simulink model "ACC_Example"  (R2015a)
settings: Solver=ode3  StartTime=0.0  StopTime=2000  FixedStep=0.02  RelTol=1e-3
undefined symbols (not defined in the file): control, data, serial
libraries: simulink x14, dspsigops x8, simulink_extras x4, instrumentlib x4, dspswit3 x1
settings Model: SimulationMode=accelerator  CovSFcnEnable=off  Creator=Owen  LastModifiedBy=VijayaKumar
settings OptimizationCC: EfficientMapNaN2IntZero=off  AccelVerboseBuild=on
settings DebuggingCC: SolverPrmCheckMsg=warning
settings HardwareCC: TargetLongLongMode=on  TargetIntDivRoundTo=Zero  TargetEndianess=LittleEndian  TargetHWDeviceType=MATLAB Host  ProdEqTarget=off
settings SFSimCC: SimCustomInitializer=initTORCSLink();  SimCustomTerminator=terminateTORCSLink();  SimUserSources=TORCSLink.c  SimBuildMode=sf_nonincremental_build  SimGenImportedTypeDefs=on
settings CodeAppCC: MaxIdLength=128
settings GRTTargetCC: CombineOutputUpdateFcns=off  GRTInterface=on

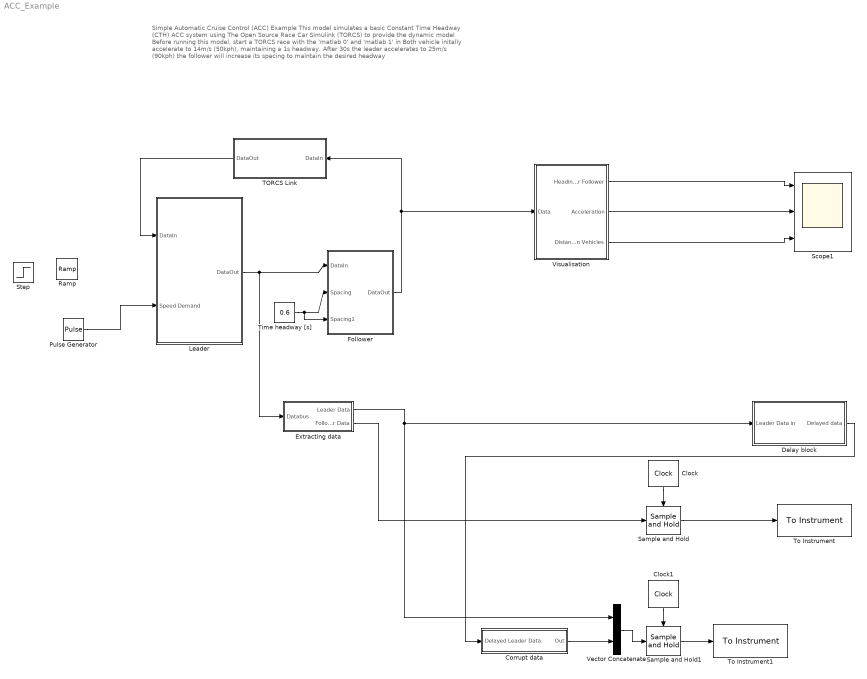
== system ACC_Example ==
  note: Simple Automatic Cruise Control (ACC) Example
      |
      | This model simulates a basic Constant Time Headway (CTH) ACC system using
      | The Open Source Race Car Simulink (TORCS) to provide the dynamic model
      |
      | Before running this model, start a TORCS race with the 'matlab 0' and 'matlab 1' in
      |
      | Both vehicle initally accelerate to 14m/s (50kph), maintaining a 1s headway.
      | After 30s the leader accelerates to 25m/s (90kph)
      | the follower will increase its spacing to maintain the desired headway
  Clock : simulink_extras/Flip Flops/Clock  period=0.04
  Clock1 : simulink_extras/Flip Flops/Clock  period=0.04
  Corrupt data : Subsystem
  "Delay block " : Subsystem
  Extracting data : Subsystem
  Follower : Subsystem
      settings: CopyFcn=|
      | veh = str2num(get_param(gcb, 'vehicle'));
      | veh = veh + 1;
      | set_param(gcb,'vehicle',num2str(veh));
  Leader : Subsystem
  Pulse Generator : DiscretePulseGenerator  PulseType=Time based  Amplitude=25  Period=60  PulseWidth=95
  Ramp : simulink/Sources/Ramp  slope=0.01  start=0  X0=15
  Sample and Hold : dspsigops/Sample and Hold  trig=Rising edge  initCond=0  latchinput=off
  Sample and Hold1 : dspsigops/Sample and Hold  trig=Rising edge  initCond=0  latchinput=off
  Scope1 : Scope  NumInputPorts=3
      settings: YMin=-0.5~-20~-2000  YMax=0.2~25~500  MaxDataPoints=30000
  Step : Step  Time=15  Before=10  After=15  SampleTime=0
  TORCS Link : Subsystem  LoadFcn=|  InitFcn=|
      LoadFcn=|
      | load VehicleBusses.mat;
      | src = 'TORCSLink.c';
      | init = 'initTORCSLink();';
      | term = 'terminateTORCSLink();';
      | simSrc = get_param(gcs,'SimUserSources');
      | simInit = get_param(gcs,'SimCustomInitializer');
      | simTerm = get_param(gcs,'SimCustomTerminator');
      | 
      | if isempty(strfind(simSrc,src))
      |   fprintf('Adding %s to Custom Sources\n', src);
      |   set_param(gcs,'SimUserSources', [simSrc 10 src]);
      | end
      | 
      | if isempty(strfind(simInit,init))
      |   fprintf('Adding %s to Custom Initialisation Code\n', init);
      |   set_param(gcs,'SimCustomInitializer', [simInit 10 init]);
      | end
      | 
      | if isempty(strfind(simTerm,term))
      |   fprintf('Adding %s to Custom Termination Code\n', term);
      |   set_param(gcs,'SimCustomTerminator', [simTerm 10 term]);
      | end
      | 
      | if isunix
      |     libs = 'librt.so';
      |     simLibs = get_param(gcs,'SimUserLibraries');
      | 
      |     if isempty(strfind(simLibs,libs))
      |       fprintf('Adding %s to Custom Libraries\n', libs);
      |       set_param(gcs,'SimUserLibraries', [simLibs 10 libs]);
      |     end
      | else
      |    set_param(gcs,'SimUserLibraries', '');
      | end
      | 
      | clear src init term simSrc simInit simTerm libs simLibs;
      InitFcn=|
      | load VehicleBusses.mat;
      | src = 'TORCSLink.c';
      | init = 'initTORCSLink();';
      | term = 'terminateTORCSLink();';
      | simSrc = get_param(gcs,'SimUserSources');
      | simInit = get_param(gcs,'SimCustomInitializer');
      | simTerm = get_param(gcs,'SimCustomTerminator');
      | 
      | if isempty(strfind(simSrc,src))
      |   fprintf('Adding %s to Custom Sources\n', src);
      |   set_param(gcs,'SimUserSources', [simSrc 10 src]);
      | end
      | 
      | if isempty(strfind(simInit,init))
      |   fprintf('Adding %s to Custom Initialisation Code\n', init);
      |   set_param(gcs,'SimCustomInitializer', [simInit 10 init]);
      | end
      | 
      | if isempty(strfind(simTerm,term))
      |   fprintf('Adding %s to Custom Termination Code\n', term);
      |   set_param(gcs,'SimCustomTerminator', [simTerm 10 term]);
      | end
      | 
      | if isunix
      |     libs = 'librt.so';
      |     simLibs = get_param(gcs,'SimUserLibraries');
      | 
      |     if isempty(strfind(simLibs,libs))
      |       fprintf('Adding %s to Custom Libraries\n', libs);
      |       set_param(gcs,'SimUserLibraries', [simLibs 10 libs]);
      |     end
      | else
      |    set_param(gcs,'SimUserLibraries', '');
      | end
      | 
      | clear src init term simSrc simInit simTerm libs simLibs;
  Time headway [s] : Constant  Value=0.6
  To Instrument : instrumentlib/To Instrument  sampleTime=-1  isWorkspaceObject=off  timeout=10  inputBufferSize=1024  protocol=Serial  serialPort=COM1  baudRate=115200  gpibVendor=Agilent Technologies  boardIndex=0  primaryAddress=1  secondaryAddress=0  visaVendor=Agilent  visaSerialPort=0  chassisIndex=0  logicalAddress=0  tcpRemoteHost='127.0.0.1'  tcpRemotePort=4500  udpRemoteHost='127.0.0.1'  udpRemotePort=9090  visaTCPBoardIndex=0  visaTCPRemoteHost='127.0.0.1'  usbBoardIndex=0  usbManufID=0  usbModelCode=0  usbSerialNumber=0  initAction=None  initCommand='DATA:SOURCE CH1'  initFunction=get  command=''  sendFormat=Binary  asciiFormatting='%d'  precision=32-bit float  byteOrder=Big Endian
  To Instrument1 : instrumentlib/To Instrument  sampleTime=-1  isWorkspaceObject=off  timeout=10  inputBufferSize=1024  protocol=Serial  serialPort=COM4  baudRate=115200  gpibVendor=Agilent Technologies  boardIndex=0  primaryAddress=1  secondaryAddress=0  visaVendor=Agilent  visaSerialPort=0  chassisIndex=0  logicalAddress=0  tcpRemoteHost='127.0.0.1'  tcpRemotePort=4500  udpRemoteHost='127.0.0.1'  udpRemotePort=9090  visaTCPBoardIndex=0  visaTCPRemoteHost='127.0.0.1'  usbBoardIndex=0  usbManufID=0  usbModelCode=0  usbSerialNumber=0  initAction=None  initCommand='DATA:SOURCE CH1'  initFunction=get  command=''  sendFormat=Binary  asciiFormatting='%d'  precision=32-bit float  byteOrder=Big Endian
  Vector Concatenate : Concatenate
  Visualisation : Subsystem
  wires:
  Leader/1(DataOut) -> Extracting data/1(Databus), Follower/1(DataIn)
  TORCS Link/1(DataOut) -> Leader/1(DataIn)
  Time headway [s]/1 -> Follower/3(Spacing1), Follower/2(Spacing)
  Clock/1 -> Sample and Hold/Trigger
  Extracting data/2(Follower Data) -> Sample and Hold/1
  Extracting data/1(Leader Data) -> Vector Concatenate/1, "Delay block "/1(Leader Data in)
  Clock1/1 -> Sample and Hold1/Trigger
  Sample and Hold1/1 -> To Instrument1/1
  Vector Concatenate/1 -> Sample and Hold1/1
  Pulse Generator/1 -> Leader/2(Speed Demand)
  Visualisation/2(Acceleration) -> Scope1/2
  Visualisation/1(Heading Error Follower) -> Scope1/1
  "Delay block "/1(Delayed data) -> Corrupt data/1(Delayed Leader Data)
  Corrupt data/1(Out) -> Vector Concatenate/2
  Follower/1(DataOut) -> TORCS Link/1(DataIn), Visualisation/1(Data)
  Visualisation/3(Distance Between Vehicles) -> Scope1/3
  Sample and Hold/1 -> To Instrument/1

== system ACC_Example/Corrupt data ==
  Delayed Leader Data : Inport
  Clock2 : simulink_extras/Flip Flops/Clock  period=0.04
  Constant{,1..3} (4 alike) : Constant  Value=2
  Counter : dspswit3/Counter  Direction=Up  CountEvent=Rising edge  CounterSize=User defined  MaxCount=255  InitialCount=0  Output=Count and Hit  HitValue=0  ResetInput=on  SamplesPerFrame=1  Ts=1  CntDtype=double  HitDtype=Logical
  "Faux Leader Data " : Concatenate  NumInputs=4
  Switch : Switch  Criteria=u2 ~= 0
  Out : Outport
  wires:
  "Faux Leader Data "/1 -> Switch/1
  Clock2/1 -> Counter/1
  Counter/2 -> Switch/2
  Constant/1 -> "Faux Leader Data "/1
  Constant1/1 -> "Faux Leader Data "/2
  Constant2/1 -> "Faux Leader Data "/3
  Constant3/1 -> "Faux Leader Data "/4
  Delayed Leader Data/1 -> Switch/3
  Switch/1 -> Out/1

== system ACC_Example/Delay block  ==
  Leader Data in : Inport
  Clock1 : simulink_extras/Flip Flops/Clock  period=0.04
  Sample & Delay 1 : dspsigops/Sample and Hold  trig=Rising edge  initCond=0  latchinput=off
  Sample & Delay {2..6} (5 alike) : dspsigops/Sample and Hold  trig=Rising edge  initCond=0  latchinput=on
  Delayed data : Outport
  wires:
  Sample & Delay 1/1 -> Sample & Delay 2/1
  Clock1/1 -> Sample & Delay 6/Trigger, Sample & Delay 5/Trigger, Sample & Delay 4/Trigger, Sample & Delay 3/Trigger, Sample & Delay 2/Trigger, Sample & Delay 1/Trigger
  Sample & Delay 2/1 -> Sample & Delay 3/1
  Sample & Delay 3/1 -> Sample & Delay 4/1
  Sample & Delay 4/1 -> Sample & Delay 5/1
  Sample & Delay 5/1 -> Sample & Delay 6/1
  Sample & Delay 6/1 -> Delayed data/1
  Leader Data in/1 -> Sample & Delay 1/1

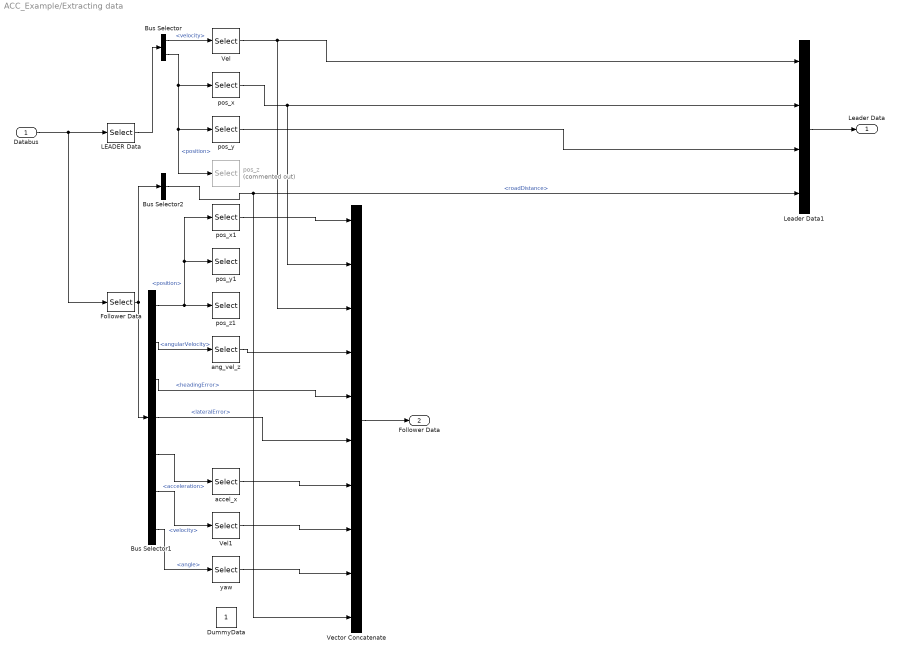
== system ACC_Example/Extracting data ==
  Databus : Inport
  Bus Selector : BusSelector  OutputSignals=data.velocity,data.position
  Bus Selector1 : BusSelector  OutputSignals=data.position,data.angularVelocity,data.headingError,data.lateralError,data.acceleration,data.velocity,data.angle
  Bus Selector2 : BusSelector  OutputSignals=data.roadDistance
  DummyData : Constant
  Follower Data : Selector  InputPortWidth=10  Indices=2
  LEADER Data : Selector  InputPortWidth=10
  Leader Data1 : Concatenate  NumInputs=4
  Vector Concatenate : Concatenate  NumInputs=10
  Vel : Selector  InputPortWidth=3
  Vel1 : Selector  InputPortWidth=3
  accel_x : Selector  InputPortWidth=3
  ang_vel_z : Selector  InputPortWidth=3  Indices=3
  pos_x : Selector  InputPortWidth=3
  pos_x1 : Selector  InputPortWidth=3
  pos_y : Selector  InputPortWidth=3  Indices=2
  pos_y1 : Selector  InputPortWidth=3  Indices=2
  pos_z : Selector  Commented=on  InputPortWidth=3  Indices=3
  pos_z1 : Selector  InputPortWidth=3  Indices=3
  yaw : Selector  InputPortWidth=3  Indices=3
  Leader Data : Outport
  Follower Data : Outport  Port=2
  wires:
  LEADER Data/1 -> Bus Selector/1
  Bus Selector/2 -> pos_z/1, pos_y/1, pos_x/1  "<position>"
  Follower Data/1 -> Bus Selector1/1, Bus Selector2/1
  Bus Selector1/2 -> ang_vel_z/1  "<angularVelocity>"
  ang_vel_z/1 -> Vector Concatenate/4
  Bus Selector1/3 -> Vector Concatenate/5  "<headingError>"
  Bus Selector1/5 -> accel_x/1  "<acceleration>"
  Bus Selector/1 -> Vel/1  "<velocity>"
  Bus Selector1/6 -> Vel1/1  "<velocity>"
  Bus Selector1/1 -> pos_x1/1, pos_y1/1, pos_z1/1  "<position>"
  Bus Selector1/7 -> yaw/1  "<angle>"
  pos_x1/1 -> Vector Concatenate/1
  accel_x/1 -> Vector Concatenate/7
  Vel1/1 -> Vector Concatenate/8
  yaw/1 -> Vector Concatenate/9
  Leader Data1/1 -> Leader Data/1
  Vector Concatenate/1 -> Follower Data/1
  Bus Selector1/4 -> Vector Concatenate/6  "<lateralError>"
  Databus/1 -> Follower Data/1, LEADER Data/1
  pos_x/1 -> Vector Concatenate/2, Leader Data1/2
  Vel/1 -> Vector Concatenate/3, Leader Data1/1
  Bus Selector2/1 -> Vector Concatenate/10, Leader Data1/4  "<roadDistance>"
  pos_y/1 -> Leader Data1/3

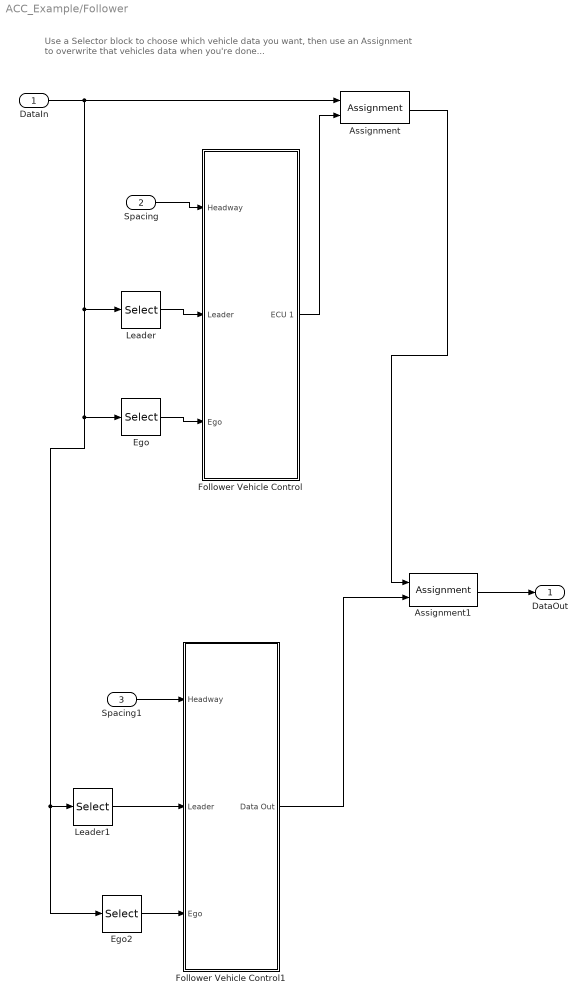
== system ACC_Example/Follower ==
  note: Use a Selector block to choose which vehicle data you want,
      | then use an Assignment to overwrite that vehicles data when you're done...
  DataIn : Inport
  Spacing : Inport  Port=2
  Spacing1 : Inport  Port=3
  Assignment : Assignment  DiagnosticForDimensions=Warning  Indices=2
  Assignment1 : Assignment  DiagnosticForDimensions=Warning  Indices=3
  Ego : Selector  InputPortWidth=10  Indices=2
  Ego2 : Selector  InputPortWidth=10  Indices=3
  Follower Vehicle Control : Subsystem
  Follower Vehicle Control1 : Subsystem
  Leader : Selector  InputPortWidth=10
  Leader1 : Selector  InputPortWidth=10
  DataOut : Outport
  wires:
  Ego/1 -> Follower Vehicle Control/3(Ego)
  DataIn/1 -> Ego2/1, Leader1/1, Ego/1, Leader/1, Assignment/1
  Spacing/1 -> Follower Vehicle Control/1(Headway)
  Leader/1 -> Follower Vehicle Control/2(Leader)
  Assignment/1 -> Assignment1/1
  Follower Vehicle Control/1(ECU 1) -> Assignment/2
  Ego2/1 -> Follower Vehicle Control1/3(Ego)
  Spacing1/1 -> Follower Vehicle Control1/1(Headway)
  Leader1/1 -> Follower Vehicle Control1/2(Leader)
  Follower Vehicle Control1/1(Data Out) -> Assignment1/2
  Assignment1/1 -> DataOut/1

== system ACC_Example/Leader ==
  note: Use a Selector block to choose which vehicle data you want,
      | then use an Assignment to overwrite that vehicles data when you're done...
  DataIn : Inport
  Speed Demand : Inport  Port=2
  Assignment : Assignment  DiagnosticForDimensions=Warning
  Lead Vehicle Control : Subsystem
  Selector : Selector  InputPortWidth=10
  DataOut : Outport
  wires:
  Speed Demand/1 -> Lead Vehicle Control/2(Speed Demand)
  DataIn/1 -> Selector/1, Assignment/1
  Selector/1 -> Lead Vehicle Control/1(Data In)
  Assignment/1 -> DataOut/1
  Lead Vehicle Control/1(Data Out) -> Assignment/2

== system ACC_Example/TORCS Link ==
  note: This subsystem handles the communicatrion with TORCS via a MATLAB function.
      | The simulation must be configured to run at a fixed sample time equal to the rate at which TORCS updates its robots (0.02s by default)
      | Data returned from TORCS is passed through a First-Order-Hold to allow continuous design in Simulink
      | Data for a maximum of 10 vehicles is returned, but not all vehicles need be present in the race
  DataIn : Inport
  FOHs : Subsystem  TreatAsAtomicUnit=on
  Memory : Memory
  Stop Simulation : Stop
  TORCSLink : MATLAB Function  TreatAsAtomicUnit=on
  DataOut : Outport
  wires:
  Memory/1 -> TORCSLink/1(vehicleDataIn)
  TORCSLink/1(vehicleDataOut) -> FOHs/1(In1)
  FOHs/1(Out1) -> DataOut/1
  DataIn/1 -> Memory/1
  TORCSLink/2(stop) -> Stop Simulation/1

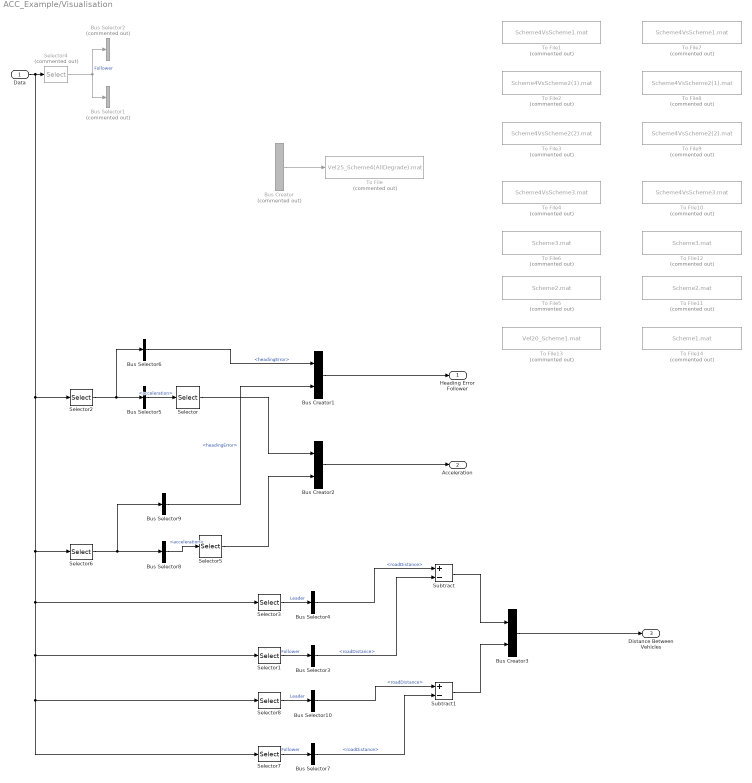
== system ACC_Example/Visualisation ==
  Data : Inport
  Bus Creator : BusCreator  Commented=on  Inputs=3
  Bus Creator1 : BusCreator  Inputs=2
  Bus Creator2 : BusCreator  Inputs=2
  Bus Creator3 : BusCreator  Inputs=2
  Bus Selector1 : BusSelector  Commented=on  OutputSignals=data.lateralError
  Bus Selector{3..4,7,10} (4 alike) : BusSelector  OutputSignals=data.roadDistance
  Bus Selector2 : BusSelector  Commented=on  OutputSignals=data.headingError
  Bus Selector5 : BusSelector  OutputSignals=data.acceleration
  Bus Selector6 : BusSelector  OutputSignals=data.headingError
  Bus Selector8 : BusSelector  OutputSignals=data.acceleration
  Bus Selector9 : BusSelector  OutputSignals=data.headingError
  Selector : Selector  InputPortWidth=3
  Selector1 : Selector  InputPortWidth=10  Indices=2
  Selector2 : Selector  InputPortWidth=10  Indices=2
  Selector3 : Selector  InputPortWidth=10
  Selector4 : Selector  Commented=on  InputPortWidth=10  Indices=2
  Selector5 : Selector  InputPortWidth=3
  Selector6 : Selector  InputPortWidth=10  Indices=3
  Selector7 : Selector  InputPortWidth=10  Indices=3
  Selector8 : Selector  InputPortWidth=10
  Subtract : Sum  Inputs=+-
  Subtract1 : Sum  Inputs=+-
  To File : ToFile  Commented=on  Filename=Vel25_Scheme4(AllDegrade).mat  SaveFormat=Timeseries
  To File1 : ToFile  Commented=on  Filename=Scheme4VsScheme1.mat  SaveFormat=Timeseries
  To File10 : ToFile  Commented=on  Filename=Scheme4VsScheme3.mat  SaveFormat=Timeseries
  To File11 : ToFile  Commented=on  Filename=Scheme2.mat  SaveFormat=Timeseries
  To File12 : ToFile  Commented=on  Filename=Scheme3.mat  SaveFormat=Timeseries
  To File13 : ToFile  Commented=on  Filename=Vel20_Scheme1.mat  SaveFormat=Timeseries
  To File14 : ToFile  Commented=on  Filename=Scheme1.mat  SaveFormat=Timeseries
  To File2 : ToFile  Commented=on  Filename=Scheme4VsScheme2(1).mat  SaveFormat=Timeseries
  To File3 : ToFile  Commented=on  Filename=Scheme4VsScheme2(2).mat  SaveFormat=Timeseries
  To File4 : ToFile  Commented=on  Filename=Scheme4VsScheme3.mat  SaveFormat=Timeseries
  To File5 : ToFile  Commented=on  Filename=Scheme2.mat  SaveFormat=Timeseries
  To File6 : ToFile  Commented=on  Filename=Scheme3.mat  SaveFormat=Timeseries
  To File7 : ToFile  Commented=on  Filename=Scheme4VsScheme1.mat  SaveFormat=Timeseries
  To File8 : ToFile  Commented=on  Filename=Scheme4VsScheme2(1).mat  SaveFormat=Timeseries
  To File9 : ToFile  Commented=on  Filename=Scheme4VsScheme2(2).mat  SaveFormat=Timeseries
  Heading Error Follower : Outport
  Acceleration : Outport  Port=2
  Distance Between Vehicles : Outport  Port=3
  wires:
  Selector4/1 -> Bus Selector2/1, Bus Selector1/1  "Follower"
  Bus Creator/1 -> To File/1
  Selector2/1 -> Bus Selector6/1, Bus Selector5/1
  Bus Selector6/1 -> Bus Creator1/1  "<headingError>"
  Bus Selector9/1 -> Bus Creator1/2  "<headingError>"
  Bus Creator1/1 -> Heading Error Follower/1
  Bus Creator2/1 -> Acceleration/1
  Bus Selector5/1 -> Selector/1  "<acceleration>"
  Selector/1 -> Bus Creator2/1
  Bus Selector8/1 -> Selector5/1  "<acceleration>"
  Selector5/1 -> Bus Creator2/2
  Selector6/1 -> Bus Selector9/1, Bus Selector8/1
  Selector3/1 -> Bus Selector4/1  "Leader"
  Bus Selector4/1 -> Subtract/1  "<roadDistance>"
  Selector1/1 -> Bus Selector3/1  "Follower"
  Bus Selector3/1 -> Subtract/2  "<roadDistance>"
  Subtract/1 -> Bus Creator3/1
  Bus Creator3/1 -> Distance Between Vehicles/1
  Selector8/1 -> Bus Selector10/1  "Leader"
  Selector7/1 -> Bus Selector7/1  "Follower"
  Data/1 -> Selector8/1, Selector7/1, Selector1/1, Selector3/1, Selector6/1, Selector2/1, Selector4/1
  Bus Selector10/1 -> Subtract1/1  "<roadDistance>"
  Bus Selector7/1 -> Subtract1/2  "<roadDistance>"
  Subtract1/1 -> Bus Creator3/2

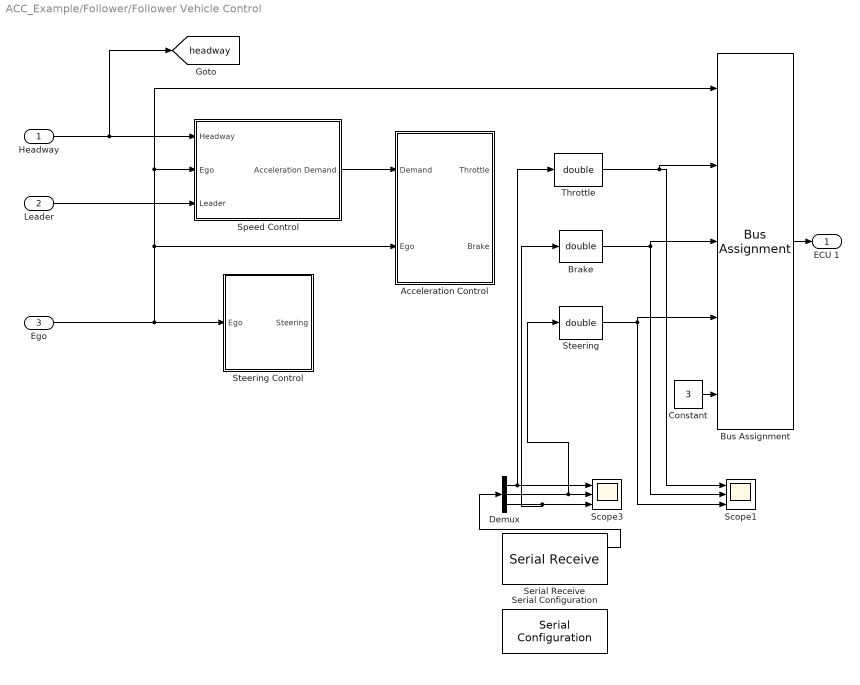
== system ACC_Example/Follower/Follower Vehicle Control ==
  Headway : Inport
  Leader : Inport  Port=2
  Ego : Inport  Port=3
  Acceleration Control : Subsystem
  Brake : DataTypeConversion  OutDataTypeStr=double
  Bus Assignment : BusAssignment  AssignedSignals=control.throttle,control.brake,control.steering,control.gear
  Constant : Constant  Value=3  OutDataTypeStr=int32
  Demux : Demux  Outputs=3
  Scope1 : Scope  NumInputPorts=3
      settings: ShowLegends=on  YMin=-0.6~-5~-5  YMax=0.6~5~5
  Scope3 : Scope  NumInputPorts=3
      settings: YMin=-3.81919~-5~-5  YMax=29.37274~5~5
  Serial Configuration : instrumentlib/Serial Configuration  Priority=-200000  ComPortMenu=<Please select a port...>  ComPort=COM2  ObjConstructor=serial('COM2');  BaudRate=115200  DataBits=8  Parity=none  StopBits=1  FlowControl=none  Timeout=10  ByteOrder=BigEndian
  Serial Receive : instrumentlib/Serial Receive  ComPortMenu=<Please select a port...>  ComPort=COM2  ObjConstructor=serial('COM2');  Terminator=<none>  DataSize="[1  3]"  DataType=single  EnableBlockingMode=off  ActionDataUnavailable=Output last received value  CustomValue=0  SampleTime=0.02
  Speed Control : Subsystem
  Steering : DataTypeConversion  OutDataTypeStr=double
  Steering Control : Subsystem
  Throttle : DataTypeConversion  OutDataTypeStr=double
  ECU 1 : Outport
  tag scope: headway=global
  wires:
  Bus Assignment/1 -> ECU 1/1
  Speed Control/1(Acceleration Demand) -> Acceleration Control/1(Demand)
  Headway/1 -> [headway], Speed Control/1(Headway)
  Ego/1 -> Bus Assignment/1, Speed Control/2(Ego), Acceleration Control/2(Ego), Steering Control/1(Ego)
  Leader/1 -> Speed Control/3(Leader)
  Constant/1 -> Bus Assignment/5
  Serial Receive/1 -> Demux/1
  Demux/1 -> Throttle/1, Scope3/1
  Demux/2 -> Steering/1, Scope3/2
  Demux/3 -> Brake/1, Scope3/3
  Throttle/1 -> Bus Assignment/2, Scope1/1
  Brake/1 -> Scope1/2, Bus Assignment/3
  Steering/1 -> Scope1/3, Bus Assignment/4

== system ACC_Example/Follower/Follower Vehicle Control1 ==
  Headway : Inport
  Leader : Inport  Port=2
  Ego : Inport  Port=3
  Acceleration Control : Subsystem
  Bus Assignment : BusAssignment  AssignedSignals=control.throttle,control.brake,control.steering,control.gear
  Constant : Constant  Value=3  OutDataTypeStr=int32
  Speed Control : Subsystem
  Steering Control : Subsystem
  Data Out : Outport
  tag scope: headway1=global
  wires:
  Bus Assignment/1 -> Data Out/1
  Speed Control/1(Acceleration Demand) -> Acceleration Control/1(Demand)
  Headway/1 -> [headway1], Speed Control/1(Headway)
  Ego/1 -> Bus Assignment/1, Speed Control/2(Ego), Acceleration Control/2(Ego), Steering Control/1(Ego)
  Leader/1 -> Speed Control/3(Leader)
  Constant/1 -> Bus Assignment/5
  Acceleration Control/1(Throttle) -> Bus Assignment/2
  Acceleration Control/2(Brake) -> Bus Assignment/3
  Steering Control/1(Steering) -> Bus Assignment/4  "steering"

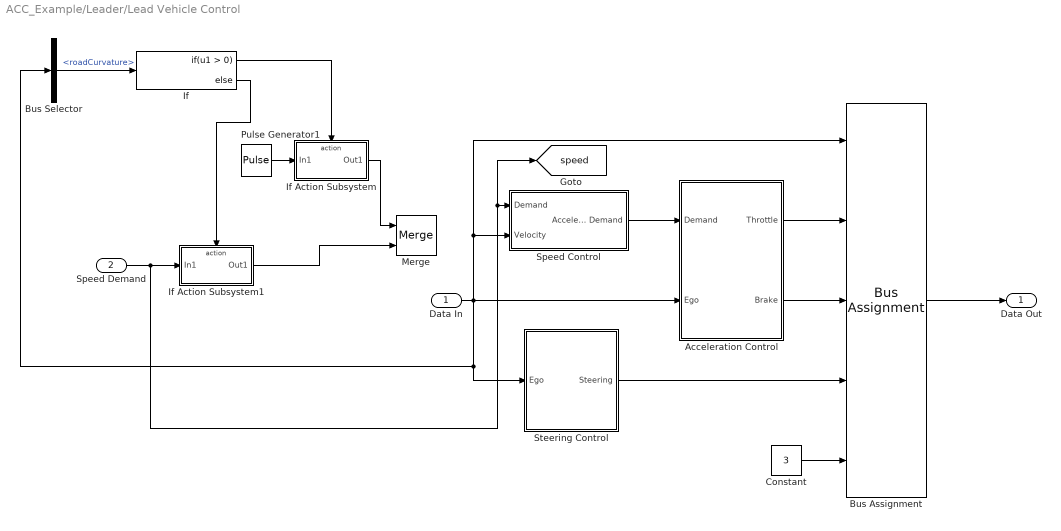
== system ACC_Example/Leader/Lead Vehicle Control ==
  Data In : Inport
  Speed Demand : Inport  Port=2
  Acceleration Control : Subsystem
  Bus Assignment : BusAssignment  AssignedSignals=control.throttle,control.brake,control.steering,control.gear
  Bus Selector : BusSelector  OutputSignals=data.roadCurvature
  Constant : Constant  Value=3  OutDataTypeStr=int32
  If : If
  If Action Subsystem : Subsystem  TreatAsAtomicUnit=on
  If Action Subsystem1 : Subsystem  TreatAsAtomicUnit=on
  Merge : Merge
  Pulse Generator1 : DiscretePulseGenerator  PulseType=Time based  Amplitude=15  Period=20  PulseWidth=85
  Speed Control : Subsystem
  Steering Control : Subsystem
  Data Out : Outport
  tag scope: speed=global
  wires:
  Bus Assignment/1 -> Data Out/1
  Speed Control/1(Acceleration Demand) -> Acceleration Control/1(Demand)
  Data In/1 -> Bus Selector/1, Steering Control/1(Ego), Bus Assignment/1, Speed Control/2(Velocity), Acceleration Control/2(Ego)
  Acceleration Control/2(Brake) -> Bus Assignment/3
  Acceleration Control/1(Throttle) -> Bus Assignment/2
  Steering Control/1(Steering) -> Bus Assignment/4
  Constant/1 -> Bus Assignment/5
  Bus Selector/1 -> If/1  "<roadCurvature>"
  If/1 -> If Action Subsystem/Action
  Pulse Generator1/1 -> If Action Subsystem/1(In1)
  If/2 -> If Action Subsystem1/Action
  If Action Subsystem/1(Out1) -> Merge/1
  If Action Subsystem1/1(Out1) -> Merge/2
  Speed Demand/1 -> Speed Control/1(Demand), [speed], If Action Subsystem1/1(In1)

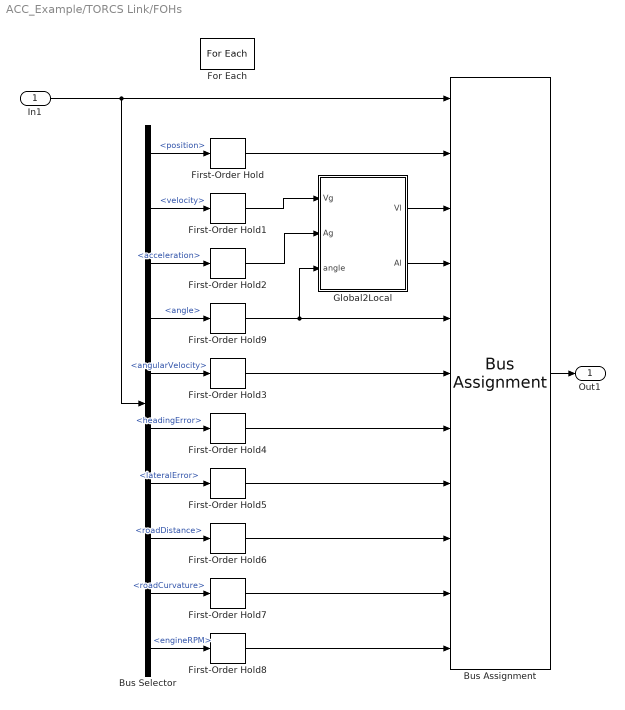
== system ACC_Example/TORCS Link/FOHs ==
  In1 : Inport  Partition=on  PartitionDimension=1  PartitionWidth=1
  Bus Assignment : BusAssignment  AssignedSignals=data.position,data.velocity,data.acceleration,data.angle,data.angularVelocity,data.headingError,data.lateralError,data.roadDistance,data.roadCurvature,data.engineRPM
  Bus Selector : BusSelector  OutputSignals=data.position,data.velocity,data.acceleration,data.angle,data.angularVelocity,data.headingError,data.lateralError,data.roadDistance,data.roadCurvature,data.engineRPM
  First-Order Hold{,1..9} (10 alike) : simulink/Discrete/First-Order Hold  DisableCoverage=on  Ts=0.02
  For Each : ForEach  DisableCoverage=on  IndexMode=One-based
  Global2Local : MATLAB Function  TreatAsAtomicUnit=on
  Out1 : Outport  ConcatenationDimension=1
  wires:
  Bus Assignment/1 -> Out1/1
  Bus Selector/10 -> First-Order Hold8/1  "<engineRPM>"
  Bus Selector/9 -> First-Order Hold7/1  "<roadCurvature>"
  Bus Selector/8 -> First-Order Hold6/1  "<roadDistance>"
  Bus Selector/7 -> First-Order Hold5/1  "<lateralError>"
  Bus Selector/6 -> First-Order Hold4/1  "<headingError>"
  Bus Selector/5 -> First-Order Hold3/1  "<angularVelocity>"
  Bus Selector/3 -> First-Order Hold2/1  "<acceleration>"
  Bus Selector/2 -> First-Order Hold1/1  "<velocity>"
  Bus Selector/1 -> First-Order Hold/1  "<position>"
  In1/1 -> Bus Assignment/1, Bus Selector/1
  Bus Selector/4 -> First-Order Hold9/1  "<angle>"
  First-Order Hold9/1 -> Global2Local/3(angle), Bus Assignment/5
  First-Order Hold3/1 -> Bus Assignment/6
  First-Order Hold4/1 -> Bus Assignment/7
  First-Order Hold5/1 -> Bus Assignment/8
  First-Order Hold6/1 -> Bus Assignment/9
  First-Order Hold7/1 -> Bus Assignment/10
  First-Order Hold8/1 -> Bus Assignment/11
  First-Order Hold1/1 -> Global2Local/1(Vg)
  First-Order Hold2/1 -> Global2Local/2(Ag)
  First-Order Hold/1 -> Bus Assignment/2
  Global2Local/2(Al) -> Bus Assignment/4
  Global2Local/1(Vl) -> Bus Assignment/3

== system ACC_Example/Follower/Follower Vehicle Control/Acceleration Control ==
  Demand : Inport
  Ego : Inport  Port=2
  Bus Selector : BusSelector  OutputSignals=data.acceleration
  Compare To Constant : simulink/Logic and Bit Operations/Compare To Constant  relop=>=  const=-0.1  OutDataTypeStr=boolean
  Logical Operator : Logic  Operator=NOT  AllPortsSameDT=off  OutDataTypeStr=boolean
  Selector : Selector  InputPortWidth=3
  Subsystem : Subsystem
  Subsystem1 : Subsystem
  Throttle : Outport
  Brake : Outport  Port=2
  wires:
  Selector/1 -> Subsystem/2(Acceleration), Subsystem1/2(Acceleration)
  Demand/1 -> Compare To Constant/1, Subsystem1/1(Demand), Subsystem/1(Demand)
  Subsystem/1(Throttle) -> Throttle/1
  Compare To Constant/1 -> Subsystem/Enable, Logical Operator/1
  Logical Operator/1 -> Subsystem1/Enable
  Ego/1 -> Bus Selector/1
  Bus Selector/1 -> Selector/1  "<acceleration>"
  Subsystem1/1(Brake) -> Brake/1

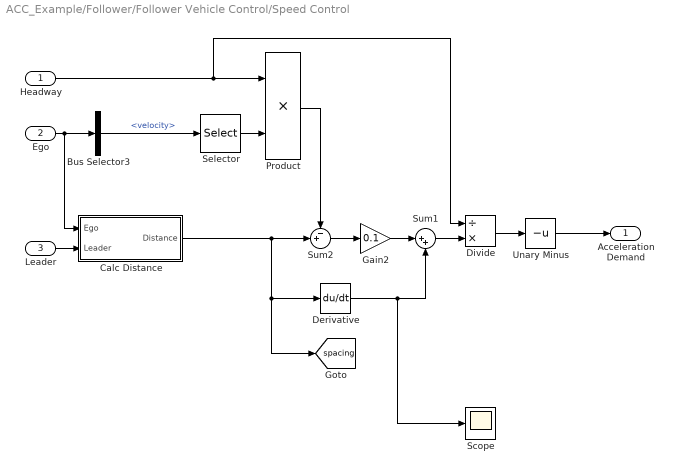
== system ACC_Example/Follower/Follower Vehicle Control/Speed Control ==
  Headway : Inport
  Ego : Inport  Port=2
  Leader : Inport  Port=3
  Bus Selector3 : BusSelector  OutputSignals=data.velocity
  Calc Distance : Subsystem
  Derivative : Derivative
  Divide : Product  Inputs=/*
  Gain2 : Gain  Gain=0.1
  Product : Product
  Scope : Scope
      settings: YMin=-52.83291  YMax=58.13725
  Selector : Selector  InputPortWidth=3
  Sum1 : Sum  Inputs=|++
  Sum2 : Sum  Inputs=-+|
  Unary Minus : UnaryMinus
  Acceleration Demand : Outport
  tag scope: spacing=global
  wires:
  Ego/1 -> Calc Distance/1(Ego), Bus Selector3/1
  Leader/1 -> Calc Distance/2(Leader)
  Headway/1 -> Divide/1, Product/1
  Selector/1 -> Product/2
  Calc Distance/1(Distance) -> Derivative/1, [spacing], Sum2/2
  Sum2/1 -> Gain2/1
  Sum1/1 -> Divide/2
  Divide/1 -> Unary Minus/1
  Unary Minus/1 -> Acceleration Demand/1
  Bus Selector3/1 -> Selector/1  "<velocity>"
  Derivative/1 -> Scope/1, Sum1/2
  Gain2/1 -> Sum1/1
  Product/1 -> Sum2/1

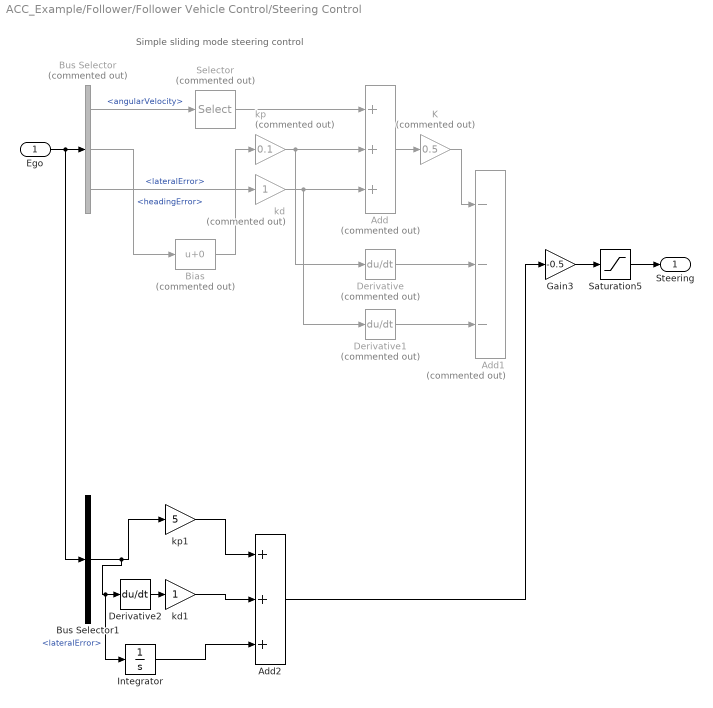
== system ACC_Example/Follower/Follower Vehicle Control/Steering Control ==
  note: Simple sliding mode steering control
  Ego : Inport
  Add : Sum  Commented=on  Inputs=+++
  Add1 : Sum  Commented=on  Inputs=---
  Add2 : Sum  Inputs=+++
  Bias : Bias  Commented=on
  Bus Selector : BusSelector  Commented=on  OutputSignals=data.angularVelocity,data.headingError,data.lateralError
  Bus Selector1 : BusSelector  OutputSignals=data.lateralError
  Derivative : Derivative  Commented=on
  Derivative1 : Derivative  Commented=on
  Derivative2 : Derivative
  Gain3 : Gain  Gain=-0.5
  Integrator : Integrator
  K : Gain  Commented=on  Gain=0.5
  Saturation5 : Saturate
  Selector : Selector  Commented=on  InputPortWidth=3  Indices=3
  kd : Gain  Commented=on
  kd1 : Gain
  kp : Gain  Commented=on  Gain=0.1
  kp1 : Gain  Gain=5
  Steering : Outport
  wires:
  Ego/1 -> Bus Selector1/1, Bus Selector/1
  K/1 -> Add1/1
  Derivative1/1 -> Add1/3
  Derivative/1 -> Add1/2
  Add/1 -> K/1
  kp/1 -> Derivative/1, Add/2
  kd/1 -> Derivative1/1, Add/3
  Bus Selector/3 -> kd/1  "<lateralError>"
  Gain3/1 -> Saturation5/1
  Saturation5/1 -> Steering/1
  Selector/1 -> Add/1
  Bus Selector/1 -> Selector/1  "<angularVelocity>"
  Bus Selector/2 -> Bias/1  "<headingError>"
  Bias/1 -> kp/1
  Bus Selector1/1 -> Integrator/1, Derivative2/1, kp1/1  "<lateralError>"
  kp1/1 -> Add2/1
  kd1/1 -> Add2/2
  Add2/1 -> Gain3/1
  Derivative2/1 -> kd1/1
  Integrator/1 -> Add2/3

== system ACC_Example/Follower/Follower Vehicle Control1/Acceleration Control ==
  Demand : Inport
  Ego : Inport  Port=2
  Bus Selector : BusSelector  OutputSignals=data.acceleration
  Compare To Constant : simulink/Logic and Bit Operations/Compare To Constant  relop=>=  const=-0.1  OutDataTypeStr=boolean
  Logical Operator : Logic  Operator=NOT  AllPortsSameDT=off  OutDataTypeStr=boolean
  Selector : Selector  InputPortWidth=3
  Subsystem : Subsystem
  Subsystem1 : Subsystem
  Throttle : Outport
  Brake : Outport  Port=2
  wires:
  Selector/1 -> Subsystem/2(Acceleration), Subsystem1/2(Acceleration)
  Demand/1 -> Compare To Constant/1, Subsystem1/1(Demand), Subsystem/1(Demand)
  Subsystem/1(Throttle) -> Throttle/1
  Compare To Constant/1 -> Subsystem/Enable, Logical Operator/1
  Logical Operator/1 -> Subsystem1/Enable
  Ego/1 -> Bus Selector/1
  Bus Selector/1 -> Selector/1  "<acceleration>"
  Subsystem1/1(Brake) -> Brake/1

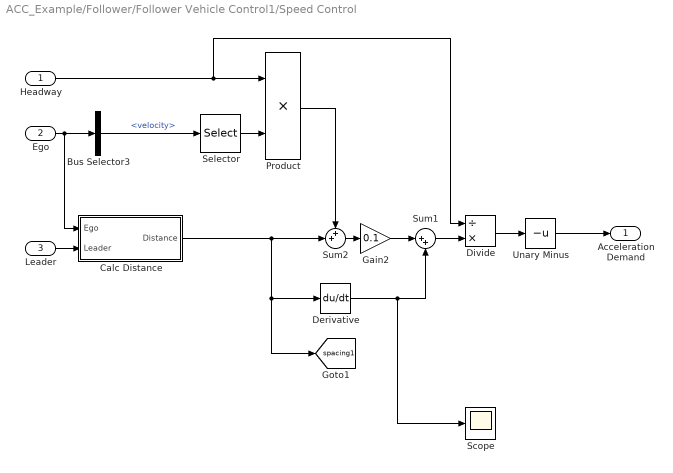
== system ACC_Example/Follower/Follower Vehicle Control1/Speed Control ==
  Headway : Inport
  Ego : Inport  Port=2
  Leader : Inport  Port=3
  Bus Selector3 : BusSelector  OutputSignals=data.velocity
  Calc Distance : Subsystem
  Derivative : Derivative
  Divide : Product  Inputs=/*
  Gain2 : Gain  Gain=0.1
  Product : Product
  Scope : Scope
      settings: YMin=-52.83291  YMax=58.13725
  Selector : Selector  InputPortWidth=3
  Sum1 : Sum  Inputs=|++
  Sum2 : Sum  Inputs=++|
  Unary Minus : UnaryMinus
  Acceleration Demand : Outport
  tag scope: spacing1=global
  wires:
  Ego/1 -> Calc Distance/1(Ego), Bus Selector3/1
  Leader/1 -> Calc Distance/2(Leader)
  Headway/1 -> Divide/1, Product/1
  Selector/1 -> Product/2
  Calc Distance/1(Distance) -> Derivative/1, [spacing1], Sum2/2
  Product/1 -> Sum2/1
  Sum2/1 -> Gain2/1
  Gain2/1 -> Sum1/1
  Sum1/1 -> Divide/2
  Divide/1 -> Unary Minus/1
  Unary Minus/1 -> Acceleration Demand/1
  Bus Selector3/1 -> Selector/1  "<velocity>"
  Derivative/1 -> Scope/1, Sum1/2

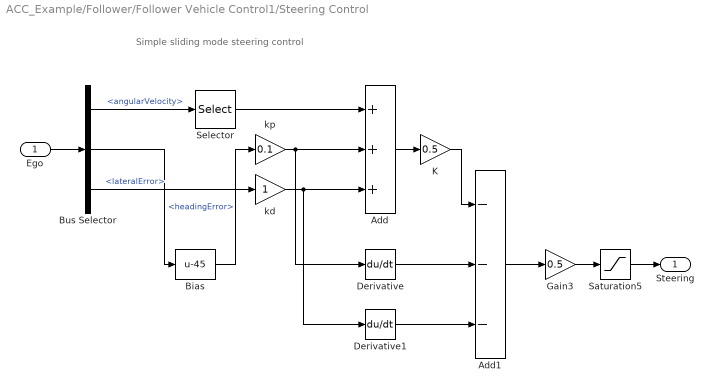
== system ACC_Example/Follower/Follower Vehicle Control1/Steering Control ==
  note: Simple sliding mode steering control
  Ego : Inport
  Add : Sum  Inputs=+++
  Add1 : Sum  Inputs=---
  Bias : Bias  Bias=-45
  Bus Selector : BusSelector  OutputSignals=data.angularVelocity,data.headingError,data.lateralError
  Derivative : Derivative
  Derivative1 : Derivative
  Gain3 : Gain  Gain=0.5
  K : Gain  Gain=0.5
  Saturation5 : Saturate
  Selector : Selector  InputPortWidth=3  Indices=3
  kd : Gain
  kp : Gain  Gain=0.1
  Steering : Outport
  wires:
  Ego/1 -> Bus Selector/1
  Add1/1 -> Gain3/1
  K/1 -> Add1/1
  Derivative1/1 -> Add1/3
  Derivative/1 -> Add1/2
  Add/1 -> K/1
  kp/1 -> Derivative/1, Add/2
  kd/1 -> Derivative1/1, Add/3
  Bus Selector/3 -> kd/1  "<lateralError>"
  Bus Selector/2 -> Bias/1  "<headingError>"
  Gain3/1 -> Saturation5/1
  Saturation5/1 -> Steering/1
  Selector/1 -> Add/1
  Bus Selector/1 -> Selector/1  "<angularVelocity>"
  Bias/1 -> kp/1

== system ACC_Example/Leader/Lead Vehicle Control/Acceleration Control ==
  Demand : Inport
  Ego : Inport  Port=2
  Bus Selector : BusSelector  OutputSignals=data.acceleration
  Compare To Constant : simulink/Logic and Bit Operations/Compare To Constant  relop=>=  const=-0.1  OutDataTypeStr=boolean
  Logical Operator : Logic  Operator=NOT  AllPortsSameDT=off  OutDataTypeStr=boolean
  Selector : Selector  InputPortWidth=3
  Subsystem : Subsystem
  Subsystem1 : Subsystem
  Throttle : Outport
  Brake : Outport  Port=2
  wires:
  Selector/1 -> Subsystem/2(Acceleration), Subsystem1/2(Acceleration)
  Demand/1 -> Compare To Constant/1, Subsystem1/1(Demand), Subsystem/1(Demand)
  Subsystem1/1(Brake) -> Brake/1
  Subsystem/1(Throttle) -> Throttle/1
  Compare To Constant/1 -> Subsystem/Enable, Logical Operator/1
  Logical Operator/1 -> Subsystem1/Enable
  Ego/1 -> Bus Selector/1
  Bus Selector/1 -> Selector/1  "<acceleration>"

== system ACC_Example/Leader/Lead Vehicle Control/If Action Subsystem ==
  In1 : Inport
  Action Port : ActionPort  ActionType=then
  Out1 : Outport
  wires:
  In1/1 -> Out1/1

== system ACC_Example/Leader/Lead Vehicle Control/If Action Subsystem1 ==
  In1 : Inport
  Action Port : ActionPort  ActionType=else
  Out1 : Outport
  wires:
  In1/1 -> Out1/1

== system ACC_Example/Leader/Lead Vehicle Control/Speed Control ==
  Demand : Inport
  Velocity : Inport  Port=2
  Bus Selector : BusSelector  OutputSignals=data.velocity
  Gain : Gain  Gain=0.5
  Rate Limiter : RateLimiter  RisingSlewLimit=inf  FallingSlewLimit=-inf  SampleTimeMode=inherited
  Saturation : Saturate  UpperLimit=2  LowerLimit=-4
  Selector : Selector  InputPortWidth=3
  Sum : Sum  Inputs=|+-
  Acceleration Demand : Outport
  wires:
  Gain/1 -> Saturation/1
  Sum/1 -> Gain/1
  Demand/1 -> Sum/1
  Saturation/1 -> Rate Limiter/1
  Selector/1 -> Sum/2
  Rate Limiter/1 -> Acceleration Demand/1
  Velocity/1 -> Bus Selector/1
  Bus Selector/1 -> Selector/1  "<velocity>"

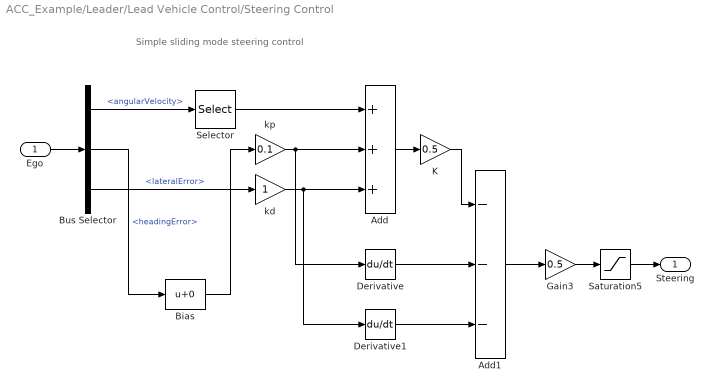
== system ACC_Example/Leader/Lead Vehicle Control/Steering Control ==
  note: Simple sliding mode steering control
  Ego : Inport
  Add : Sum  Inputs=+++
  Add1 : Sum  Inputs=---
  Bias : Bias
  Bus Selector : BusSelector  OutputSignals=data.angularVelocity,data.headingError,data.lateralError
  Derivative : Derivative
  Derivative1 : Derivative
  Gain3 : Gain  Gain=0.5
  K : Gain  Gain=0.5
  Saturation5 : Saturate
  Selector : Selector  InputPortWidth=3  Indices=3
  kd : Gain
  kp : Gain  Gain=0.1
  Steering : Outport
  wires:
  Ego/1 -> Bus Selector/1
  Add1/1 -> Gain3/1
  K/1 -> Add1/1
  Derivative1/1 -> Add1/3
  Derivative/1 -> Add1/2
  Add/1 -> K/1
  kp/1 -> Derivative/1, Add/2
  kd/1 -> Derivative1/1, Add/3
  Bus Selector/3 -> kd/1  "<lateralError>"
  Gain3/1 -> Saturation5/1
  Saturation5/1 -> Steering/1
  Selector/1 -> Add/1
  Bus Selector/1 -> Selector/1  "<angularVelocity>"
  Bus Selector/2 -> Bias/1  "<headingError>"
  Bias/1 -> kp/1

== system ACC_Example/Follower/Follower Vehicle Control/Acceleration Control/Subsystem ==
  Demand : Inport
  Acceleration : Inport  Port=2
  Enable : EnablePort  StatesWhenEnabling=reset
  Gain : Gain  Gain=1.5
  Gain1 : Gain  Gain=10
  Integrator Limited : Integrator  LimitOutput=on  UpperSaturationLimit=1  LowerSaturationLimit=-1
  Scope : Scope  NumInputPorts=2
      settings: ShowLegends=on  YMin=-36.35325~-5  YMax=327.17922~5  SaveName=ScopeData5
  Sum : Sum  Inputs=++|
  Sum1 : Sum  Inputs=+-|
  Throttle : Outport  OutputWhenDisabled=reset  InitialOutput=0
  wires:
  Gain/1 -> Sum/1
  Integrator Limited/1 -> Scope/2, Sum/2
  Gain1/1 -> Scope/1, Integrator Limited/1
  Sum/1 -> Throttle/1
  Demand/1 -> Sum1/1
  Acceleration/1 -> Sum1/2
  Sum1/1 -> Gain/1, Gain1/1

== system ACC_Example/Follower/Follower Vehicle Control/Acceleration Control/Subsystem1 ==
  Demand : Inport
  Acceleration : Inport  Port=2
  Enable : EnablePort  StatesWhenEnabling=reset
  Gain2 : Gain  Gain=0.005
  Gain3 : Gain
  Integrator Limited : Integrator  LimitOutput=on  UpperSaturationLimit=1  LowerSaturationLimit=-1
  Saturation1 : Saturate  UpperLimit=1  LowerLimit=0
  Sum1 : Sum  Inputs=-+|
  Sum2 : Sum  Inputs=++|
  Brake : Outport  OutputWhenDisabled=reset  InitialOutput=0
  wires:
  Saturation1/1 -> Brake/1
  Sum2/1 -> Saturation1/1
  Gain2/1 -> Sum2/2
  Integrator Limited/1 -> Sum2/1
  Gain3/1 -> Integrator Limited/1
  Sum1/1 -> Gain2/1, Gain3/1
  Demand/1 -> Sum1/1
  Acceleration/1 -> Sum1/2

== system ACC_Example/Follower/Follower Vehicle Control/Speed Control/Calc Distance ==
  note: Assuming vehicles are following each other, Euclidian distance equates to separation
  Ego : Inport
  Leader : Inport  Port=2
  Bus Selector : BusSelector  OutputSignals=data.position
  Bus Selector1 : BusSelector  OutputSignals=data.position
  Car Length : Constant  Value=5
  Math Function : Math  Operator=square  SaturateOnIntegerOverflow=on
  Sqrt : Sqrt  SaturateOnIntegerOverflow=on
  Sum : Sum  Inputs=|+-
  Sum of Elements : Sum  Inputs=+
  Sum1 : Sum  Inputs=|-+
  Distance : Outport
  wires:
  Ego/1 -> Bus Selector/1
  Leader/1 -> Bus Selector1/1
  Bus Selector/1 -> Sum/1  "<position>"
  Bus Selector1/1 -> Sum/2  "<position>"
  Sum/1 -> Math Function/1
  Math Function/1 -> Sum of Elements/1
  Sum of Elements/1 -> Sqrt/1
  Sum1/1 -> Distance/1
  Sqrt/1 -> Sum1/1
  Car Length/1 -> Sum1/2

== system ACC_Example/Follower/Follower Vehicle Control1/Acceleration Control/Subsystem ==
  Demand : Inport
  Acceleration : Inport  Port=2
  Enable : EnablePort  StatesWhenEnabling=reset
  Gain : Gain  Gain=1.5
  Gain1 : Gain  Gain=10
  Integrator Limited : Integrator  LimitOutput=on  UpperSaturationLimit=1  LowerSaturationLimit=-1
  Scope : Scope  NumInputPorts=2
      settings: ShowLegends=on  YMin=-36.35325~-5  YMax=327.17922~5  SaveName=ScopeData5
  Sum : Sum  Inputs=++|
  Sum1 : Sum  Inputs=+-|
  Throttle : Outport  OutputWhenDisabled=reset  InitialOutput=0
  wires:
  Gain/1 -> Sum/1
  Integrator Limited/1 -> Scope/2, Sum/2
  Gain1/1 -> Scope/1, Integrator Limited/1
  Sum/1 -> Throttle/1
  Demand/1 -> Sum1/1, Gain/1
  Acceleration/1 -> Sum1/2
  Sum1/1 -> Gain1/1

== system ACC_Example/Follower/Follower Vehicle Control1/Acceleration Control/Subsystem1 ==
  Demand : Inport
  Acceleration : Inport  Port=2
  Enable : EnablePort  StatesWhenEnabling=reset
  Gain2 : Gain  Gain=0.005
  Gain3 : Gain
  Integrator Limited : Integrator  LimitOutput=on  UpperSaturationLimit=1  LowerSaturationLimit=-1
  Saturation1 : Saturate  UpperLimit=1  LowerLimit=0
  Sum1 : Sum  Inputs=-+|
  Sum2 : Sum  Inputs=++|
  Brake : Outport  OutputWhenDisabled=reset  InitialOutput=0
  wires:
  Saturation1/1 -> Brake/1
  Sum2/1 -> Saturation1/1
  Gain2/1 -> Sum2/2
  Integrator Limited/1 -> Sum2/1
  Gain3/1 -> Integrator Limited/1
  Sum1/1 -> Gain2/1, Gain3/1
  Demand/1 -> Sum1/1
  Acceleration/1 -> Sum1/2

== system ACC_Example/Follower/Follower Vehicle Control1/Speed Control/Calc Distance ==
  note: Assuming vehicles are following each other, Euclidian distance equates to separation
  Ego : Inport
  Leader : Inport  Port=2
  Bus Selector : BusSelector  OutputSignals=data.position
  Bus Selector1 : BusSelector  OutputSignals=data.position
  Car Length : Constant  Value=5
  Math Function : Math  Operator=square  SaturateOnIntegerOverflow=on
  Sqrt : Sqrt  SaturateOnIntegerOverflow=on
  Sum : Sum  Inputs=|+-
  Sum of Elements : Sum  Inputs=+
  Sum1 : Sum  Inputs=|-+
  Distance : Outport
  wires:
  Ego/1 -> Bus Selector/1
  Leader/1 -> Bus Selector1/1
  Bus Selector/1 -> Sum/1  "<position>"
  Bus Selector1/1 -> Sum/2  "<position>"
  Sum/1 -> Math Function/1
  Math Function/1 -> Sum of Elements/1
  Sum of Elements/1 -> Sqrt/1
  Sum1/1 -> Distance/1
  Sqrt/1 -> Sum1/1
  Car Length/1 -> Sum1/2

== system ACC_Example/Leader/Lead Vehicle Control/Acceleration Control/Subsystem ==
  Demand : Inport
  Acceleration : Inport  Port=2
  Enable : EnablePort  StatesWhenEnabling=reset
  Gain : Gain  Gain=1.5
  Gain1 : Gain  Gain=10
  Integrator Limited : Integrator  LimitOutput=on  UpperSaturationLimit=1  LowerSaturationLimit=-1
  Sum : Sum  Inputs=++|
  Sum1 : Sum  Inputs=+-|
  Throttle : Outport  OutputWhenDisabled=reset  InitialOutput=0
  wires:
  Gain/1 -> Sum/1
  Integrator Limited/1 -> Sum/2
  Gain1/1 -> Integrator Limited/1
  Sum/1 -> Throttle/1
  Demand/1 -> Sum1/1, Gain/1
  Acceleration/1 -> Sum1/2
  Sum1/1 -> Gain1/1

== system ACC_Example/Leader/Lead Vehicle Control/Acceleration Control/Subsystem1 ==
  Demand : Inport
  Acceleration : Inport  Port=2
  Enable : EnablePort  StatesWhenEnabling=reset
  Gain2 : Gain  Gain=0.005
  Gain3 : Gain
  Integrator Limited : Integrator  LimitOutput=on  UpperSaturationLimit=1  LowerSaturationLimit=-1
  Saturation1 : Saturate  UpperLimit=1  LowerLimit=0
  Sum1 : Sum  Inputs=-+|
  Sum2 : Sum  Inputs=++|
  Brake : Outport  OutputWhenDisabled=reset  InitialOutput=0
  wires:
  Saturation1/1 -> Brake/1
  Sum2/1 -> Saturation1/1
  Gain2/1 -> Sum2/2
  Integrator Limited/1 -> Sum2/1
  Gain3/1 -> Integrator Limited/1
  Sum1/1 -> Gain2/1, Gain3/1
  Demand/1 -> Sum1/1
  Acceleration/1 -> Sum1/2

== matlab function ACC_Example/TORCS Link/TORCSLink ==
  data: vehicleDataIn input Bus: VehicleBus size=10; vehicleDataOut output Bus: VehicleBus size=10; stop output
function [vehicleDataOut, stop] = TORCSLink(vehicleDataIn)
%#codegen
stop = 0;
flag = int32(0);

% Simulink doesn't like passing the array of structures to C function (no
% idea why?!), so we have to seperate out the three stages

% Update vehicle control values in TORCS
for i=1:10
    flag = coder.ceval('setVehicleControl', int32(i-1), vehicleDataIn(i).control);
    if (flag < 0)
        fprintf('No connection to TORCS!\n');
        stop = 1;
    end
end

% Tell TORCS it can update (this function hangs until new data is
% available)
flag = coder.ceval('updateTORCS');
if (flag < 0)
    fprintf('No data from TORCS! (%d) \n', flag);
    stop = 1;
end

% Read in new data from TORCS
for i=1:10
    % Can't pass this directly to coder.ref
    data = vehicleDataIn(i).data;
    flag = coder.ceval('getVehicleData', int32(i-1), coder.ref(data));
    vehicleDataIn(i).data = data;
    if (flag < 0)
        fprintf('No connection to TORCS!\n');
        stop = 1;
    end
end

vehicleDataOut = vehicleDataIn;

== matlab function ACC_Example/TORCS Link/FOHs/Global2Local ==
  data: Vg input; Ag input; angle input; Vl output; Al output
function [Vl,Al] = fcn(Vg,Ag,angle)
%#codegen

phi=angle(3);
R = [cos(phi) sin(phi) 0; -sin(phi) cos(phi) 0; 0 0 1];

Vl = R*Vg;
Al = R*Ag;
